simulink model "XY_2mm_accelcontrol"  (R2023a)
settings: Solver=ode1  StartTime=0.0  StopTime=inf  FixedStep=0.001  RelTol=1e-3  EnableMultiTasking=on
PostLoadFcn:
  | , if any(exist('dsrtsu_mdlpostloadfcn', 'file') ~= 0), dsrtsu_mdlpostloadfcn('Execute', bdroot); end,
InitFcn:
  | , if any(exist('rtifpga_mdlclblib', 'file') ~= 0), rtifpga_mdlclblib('Init', bdroot); end,
  | [b,a] = butter(6,0.6)
  | N_coils = 6
  | % Load mean voltage needed for stationary levitation at "center" for the ML model's given dataset
  | load("D:\Maglev_Project\00_WORKSTATION\MATLAB Training\alldata.mat","Vmean_raw")
  | tic
model workspace (MAT data in the model file):
  Iters = 5
  N_coils = 6
  fatness_default = 1
  running = 0
  z0_default = 0.080001
undefined symbols (not defined in the file or in its folder): a, b, DiscIntNeverNeededParam, Vmean_raw
libraries: neural x15, simulink x8, commfilt2 x7, dspstat3 x4, rti2004lib x3, rtilibm x1
(part 3 of 3)

== matlab function XY_2mm_accelcontrol/get_plant_input/choose_Z_d_temp/choose_Zd_temp ==
  data: Z_d input; Z_d_temp output; z input; z_mean input; smooth_levitation_params input; recovery_mode input
function Z_d_temp = choose_Zd_temp(Z_d, z, z_mean, smooth_levitation_params, recovery_mode)
    dz = Z_d - z;
    
    % Choose maximum |dz| based on recovery mode
    if recovery_mode==0
        % 'safe'
        dz_max = smooth_levitation_params(1);
    elseif recovery_mode==1
        % 'panic'
        dz_max = 0;
    elseif recovery_mode==2
        % 'recovery'
        dz_max = smooth_levitation_params(2);
    else
        % There is no other recovery mode.
        dz_max = smooth_levitation_params(1);
    end

    % Enforce dz_max.
    if abs(dz) > dz_max
        Z_d_temp = z_mean + sign(dz)*dz_max;
    else
        % Z is within the acceptable distance from Z_d, so do nothing!
        Z_d_temp = Z_d;
    end

== matlab function XY_2mm_accelcontrol/Monitoring/diagnostics ==
  data: magnet_specs output; magnet_specs input; xyz input; signal_raw input; h123_off_minmax input; h123_empty_minmax input; z_rest_minmax input; h1_off output; h2_off output; h3_off output; h1_empty output; h2_or_h3_empty output; z_resting output; z_resting_too_low output; in_workspace output
function [magnet_specs, h1_off, h2_off, h3_off, h1_empty, h2_or_h3_empty, z_resting, z_resting_too_low, in_workspace] = get_status(magnet_specs, xyz, signal_raw, h123_off_minmax, h123_empty_minmax, z_rest_minmax)
% Detects state of the magnet and/or laser sensors based on position data.
% Assumes that the values thresholds (i.e. inputs, such as h123_off_minmax)
% have already been calibrated beforehand.
%
% The resulting ``status" can then be read by ControlDesk and/or Python.
%
%   States:
%   -------
%   0 : "off" (Laser sensors are likely turned off.)
%   1 : "rest" (Magnet is resting on top of the platform.)
%   1.01: "rest-too-low" (magnet is somehow below a height of zero)
%   1.1 : "rest-short" (Magnet is resting on top of the platform, but is
%          too short for X, Y to be detected.)
%   1.11 : "rest-short-too-low" (Magnet is somehow below a height of zero,
%          and is too short for X, Y to be detected.)
%   2 : "levitating" (Magnet is levitating at some X, Y, Z position.)
%   2.1 : "levitating-short" (Magnet is levitating, but too low/high for X,
%          Y to be detected.)
%   2.2 : "levitating-offside" (Magnet is levitating, but Z is not detected
%          while X, Y are.)
%   9 : "empty" (Empty platform detected; magnet has left workspace.)
%   10 : "true_empty" (Everything is absent, including the platform. Should
%          never happen.)
%   999 : "other" (None of the above. Should never happen.)
    height_m = magnet_specs(2);
    x = xyz(1);
    y = xyz(2);
    z = xyz(3);
    head1_raw = signal_raw(1);
    head2_raw = signal_raw(2); % (sic)
    head3_raw = signal_raw(3); % (sic)

    h1_off_min = min(h123_off_minmax(1:2));
    h1_off_max = max(h123_off_minmax(1:2));
    h2_off_min = min(h123_off_minmax(3:4));
    h2_off_max = max(h123_off_minmax(3:4));
    h3_off_min = min(h123_off_minmax(5:6));
    h3_off_max = max(h123_off_minmax(5:6));

    h1_empty_min = min(h123_empty_minmax(1:2));
    h1_empty_max = max(h123_empty_minmax(1:2));
    h2_empty_min = min(h123_empty_minmax(3:4));
    h2_empty_max = max(h123_empty_minmax(3:4));
    h3_empty_min = min(h123_empty_minmax(5:6));
    h3_empty_max = max(h123_empty_minmax(4:6));

    % Detect on/off/empty/etc for each reading
    h1_off = head1_raw > h1_off_min && head1_raw < h1_off_max;
    h2_off = head2_raw > h2_off_min && head2_raw < h2_off_max;
    h3_off = head3_raw > h3_off_min && head3_raw < h3_off_max;

    h1_empty = head1_raw > h1_empty_min && head1_raw < h1_empty_max;
    h2_empty = head2_raw > h2_empty_min && head2_raw < h2_empty_max;
    h3_empty = head3_raw > h3_empty_min && head3_raw < h3_empty_max;
    h2_or_h3_empty = h2_empty || h3_empty;
    
    % Detect resting / levitating / etc
    z_rest_min = min(z_rest_minmax);
    z_rest_max = max(z_rest_minmax);
    z_resting = z > z_rest_min && z < z_rest_max;
    z_resting_too_low = z <= z_rest_min && z < z_rest_max ...
                  && z > -height_m && ~h1_empty;
    in_workspace =   ~(h1_off   && h2_off   && h3_off) ...
                  && ~(h1_empty && h2_empty && h3_empty) ...
                  && (z > -height_m);

== matlab function XY_2mm_accelcontrol/Monitoring/diagnostics_summary ==
  data: h1_off input; h2_off input; h3_off input; h1_empty input; h2_or_h3_empty input; z_resting input; z_resting_too_low input; in_workspace input; z_stable input; z_converged input; fully_off output; resting output; empty_workspace output; recording_safe output; e_stop input
function [fully_off, resting, empty_workspace, recording_safe] = summarize_status(h1_off, h2_off, h3_off, h1_empty, h2_or_h3_empty, z_resting, z_resting_too_low, in_workspace, z_stable, z_converged, e_stop)
% 
%     - are sensors off?
%     - is magnet resting?
%         - is magnet resting below XY sensors?
%     - is workspace empty?
%     - is there reason to stop RECORDING? e.g.:
%         - X readings empty
%         - Y readings empty
%         - Z readings empty
%         - Z not converged
%         - magnet resting on platform
%         - sensors off
%         - E-stop on


    % Detect off
    % 0 - sensors on
    % 1 - sensors off
    if h1_off && h2_off && h3_off
        fully_off = 1;
    else
        fully_off = 0;
    end

    % Detect resting on the platform
    % 0 - not on platform
    % 1 - on platform
    % 2 - on platform (XY not detected)
    % 3 - on platform ((!) NONSENSICALLY LOW)
    if z_resting_too_low
        resting = 3;
    elseif z_resting && (h2_or_h3_empty)
        resting = 2;
    elseif z_resting
        resting = 1;
    else
        resting = 0;
    end

    % Detect empty workspace
    % 0 - not completely empty
    % 1 - completely empty
    empty_workspace = ~in_workspace;

    % Detect reasons to stop recording
    if h1_empty || h2_or_h3_empty ...
            || fully_off || z_resting || z_resting_too_low ...
            || ~z_converged(1) || e_stop
        recording_safe = 0;
    else
        recording_safe = 1;
    end


%     % Detect off
%     if h1_off && h2_off && h3_off
%         status = 0;
%     % Detect resting on platform (TOO LOW), but empty XY readings
%     elseif z_resting_too_low && (h2_or_h3_empty)
%         status = 1.11;
%     % Detect resting on platform, but empty XY readings
%     elseif z_resting && (h2_or_h3_empty)
%         status = 1.1;
%     % Detect resting on platform (TOO LOW)
%     elseif z_resting_too_low
%         status = 1.01;
%     % Detect resting on platform
%     elseif z_resting
%         status = 1;
%     % Detect empty reading ONLY for XY; z is still detected
%     elseif ~h1_empty && (h2_or_h3_empty)
%         status = 2.1;
%     % Detect empty reading ONLY for Z; XY still detected
%     elseif h1_empty && ~(h2_or_h3_empty)
%         status = 2.2;
%     % Detect empty reading
%     elseif h1_empty && h2_empty && h3_empty
%         status = 9;
%     % XYZ are all detected, and it's not off or empty
%     else
%         status = 2;
%     end
end
